simulink model "model_3"  (R2021b)
settings: Solver=VariableStepAuto  StartTime=0.0  StopTime=100  RelTol=1e-3
settings Model: Creator=vital  LastModifiedBy=kirba

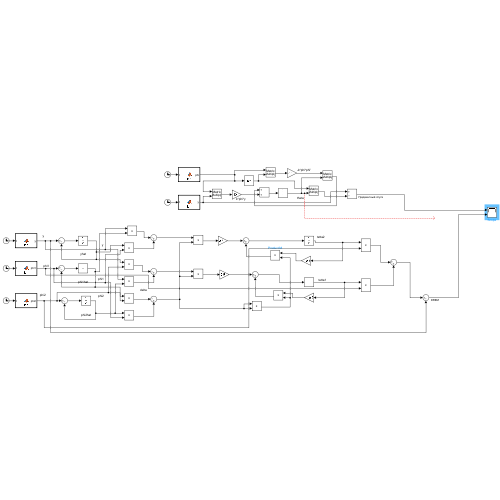
[thumbnail: Simulink's stored preview of the top-level diagram]
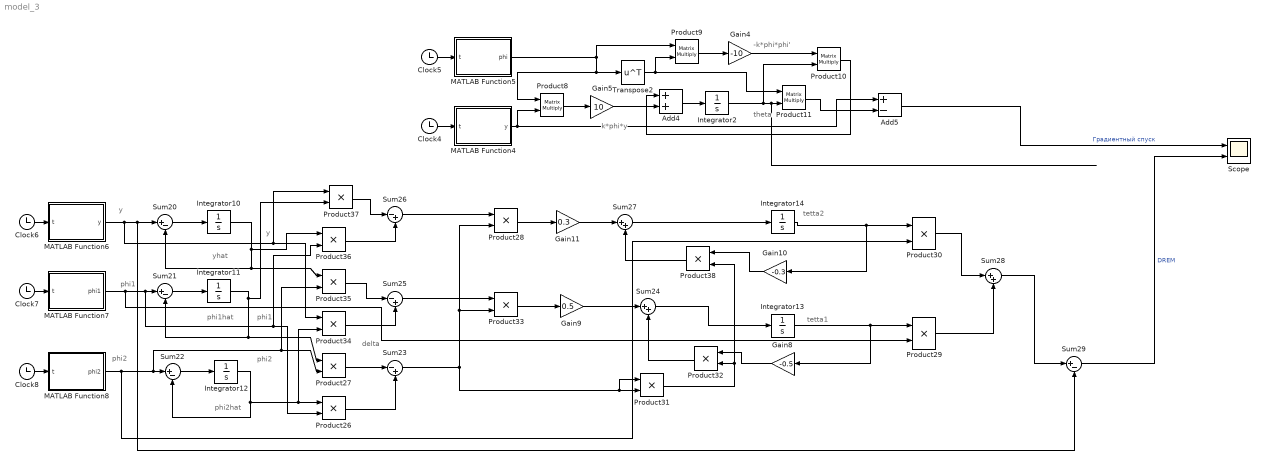
== system model_3 ==
  note: phi2
  note: phi2hat
  note: y
  note: phi1hat
  note: yhat
  note: phi1
  note: delta
  note: tetta1
  note: phi1
  note: tetta2
  note: phi2
  note: y
  note: k*phi*y
  note: -k*phi*phi'
  note: theta
  Add4 : Sum
  Add5 : Sum  Inputs=+-
  Clock{4..8} (5 alike) : Clock
  Gain10 : Gain  Gain=-0.3
  Gain11 : Gain  Gain=0.3
  Gain4 : Gain  Gain=-10
  Gain5 : Gain  Gain=10
  Gain8 : Gain  Gain=-0.5
  Gain9 : Gain  Gain=0.5
  Integrator{2,10..14} (6 alike) : Integrator
  MATLAB Function4 : MATLAB Function  TreatAsAtomicUnit=on
  MATLAB Function5 : MATLAB Function  TreatAsAtomicUnit=on
  MATLAB Function6 : MATLAB Function  TreatAsAtomicUnit=on
  MATLAB Function7 : MATLAB Function  TreatAsAtomicUnit=on
  MATLAB Function8 : MATLAB Function  TreatAsAtomicUnit=on
  Product{8..11} (4 alike) : Product  Multiplication=Matrix(*)
  Product{26..38} (13 alike) : Product
  Scope : Scope  NumInputPorts=2
  Sum{20..22,29} (4 alike) : Sum  Inputs=|+-
  Sum23 : Sum  Inputs=|-+
  Sum24 : Sum  Inputs=|++
  Sum25 : Sum  Inputs=|-+
  Sum26 : Sum  Inputs=|-+
  Sum27 : Sum  Inputs=|++
  Sum28 : Sum  Inputs=|++
  Transpose2 : Math  Operator=transpose  SaturateOnIntegerOverflow=on
  wires:
  Sum21/1 -> Integrator11/1
  Product27/1 -> Sum23/1
  Product26/1 -> Sum23/2
  Clock7/1 -> MATLAB Function7/1(t)
  Integrator10/1 -> Product35/1, Sum20/2, Product36/1
  Clock6/1 -> MATLAB Function6/1(t)
  Sum20/1 -> Integrator10/1
  MATLAB Function7/1(phi1) -> Product29/2, Product36/2, Product26/2, Sum21/1
  Sum25/1 -> Product33/1
  Product31/1 -> Product38/2, Product32/2
  Sum26/1 -> Product28/1
  Product34/1 -> Sum25/2
  Product35/1 -> Sum25/1
  Sum22/1 -> Integrator12/1
  Product32/1 -> Sum24/2
  Product36/1 -> Sum26/2
  Gain11/1 -> Sum27/1
  Product28/1 -> Gain11/1
  Integrator14/1 -> Product30/1, Gain10/1
  Sum23/1 -> Product28/2, Product33/2, Product31/1, Product31/2
  Product29/1 -> Sum28/2
  Product37/1 -> Sum26/1
  Gain8/1 -> Product32/1
  Sum28/1 -> Sum29/1
  MATLAB Function6/1(y) -> Product37/1, Product34/1, Sum29/2, Sum20/1
  Integrator12/1 -> Product34/2, Product26/1, Sum22/2
  Integrator11/1 -> Product37/2, Product27/1, Sum21/2
  Gain10/1 -> Product38/1
  Product33/1 -> Gain9/1
  Product38/1 -> Sum27/2
  Sum27/1 -> Integrator14/1
  Product30/1 -> Sum28/1
  Sum24/1 -> Integrator13/1
  MATLAB Function8/1(phi2) -> Product30/2, Product35/2, Product27/2, Sum22/1
  Clock8/1 -> MATLAB Function8/1(t)
  Gain9/1 -> Sum24/1
  Integrator13/1 -> Gain8/1, Product29/1
  MATLAB Function5/1(phi) -> Product9/1, Product8/1, Transpose2/1
  Clock4/1 -> MATLAB Function4/1(t)
  Gain4/1 -> Product10/1
  Product10/1 -> Add4/1
  Clock5/1 -> MATLAB Function5/1(t)
  Add4/1 -> Integrator2/1
  Transpose2/1 -> Product11/1, Product9/2
  Product11/1 -> Add5/2
  Product8/1 -> Gain5/1
  MATLAB Function4/1(y) -> Add5/1, Product8/2
  Product9/1 -> Gain4/1
  Gain5/1 -> Add4/2
  Integrator2/1 -> Product11/2, Product10/2
  Add5/1 -> Scope/1  "Градиентный спуск"
  Sum29/1 -> Scope/2  "DREM"

== matlab function model_3/MATLAB Function5 ==
  data: t input; phi output
function phi = fcn(t)

phi = [3*sin(t+pi/12); 5*sin(2*t)];

== matlab function model_3/MATLAB Function6 ==
  data: t input; y output
function y = fcn(t)

y = 4*3*sin(t+pi/12) +  20*5*sin(2*t);

== matlab function model_3/MATLAB Function7 ==
  data: t input; phi1 output
function phi1 = fcn(t)

phi1 = 3*sin(t+pi/12);

== matlab function model_3/MATLAB Function8 ==
  data: t input; phi2 output
function phi2 = fcn(t)

phi2 = 5*sin(2*t);

== matlab function model_3/MATLAB Function4 ==
  data: t input; y output
function y = fcn(t)

y  = 4*3*sin(t+pi/12) +  20*5*sin(2*t);
